simulink model "p10"  (R2020a)
settings: Solver=VariableStepAuto  StartTime=0.0  StopTime=10.0  RelTol=1e-3
model workspace (MAT data in the model file):
  A = 50
  Ad = 10
  B = 10
  C = 1389000
  H = 10000
  K = 2063000
  u = 1861.01
settings Model: Creator=a.kochnov  LastModifiedBy=a.kochnov

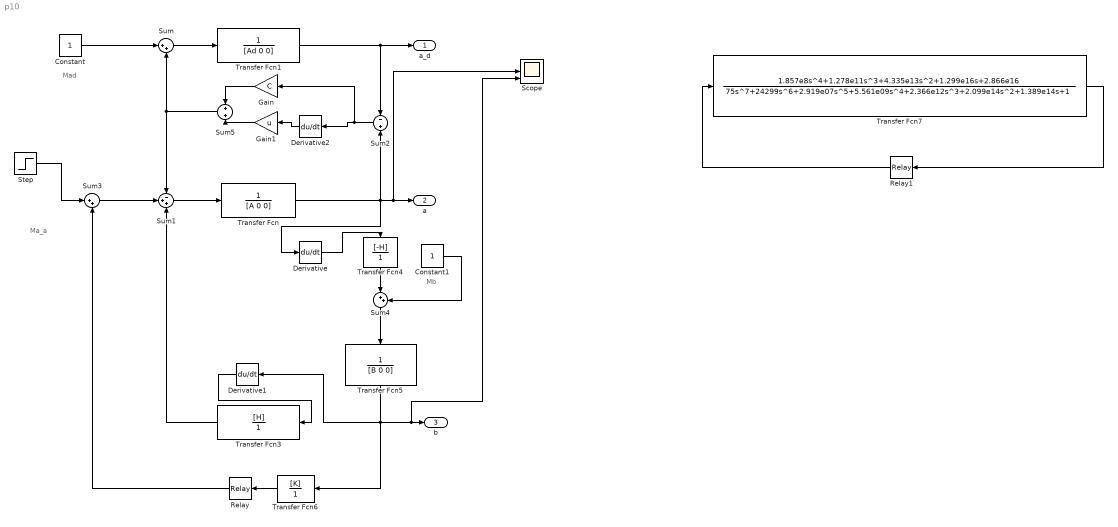
== system p10 ==
  note: Ma_a
  note: Mb
  note: Mad
  Constant : Constant
  Constant1 : Constant
  Derivative : Derivative
  Derivative1 : Derivative
  Derivative2 : Derivative
  Gain : Gain  Gain=C
  Gain1 : Gain  Gain=u
  Relay : Relay  OnSwitchValue=0  OffSwitchValue=0  OnOutputValue=10
  Relay1 : Relay  OnSwitchValue=0  OffSwitchValue=0
  Scope : Scope  NumInputPorts=3
  Step : Step  SampleTime=0
  Sum : Sum  Inputs=|++
  Sum1 : Sum  Inputs=-++
  Sum2 : Sum  Inputs=-|+
  Sum3 : Sum  Inputs=|++
  Sum4 : Sum  Inputs=|++
  Sum5 : Sum  Inputs=+|+
  Transfer Fcn : TransferFcn  Denominator=[A 0 0]
  Transfer Fcn1 : TransferFcn  Denominator=[Ad 0 0]
  Transfer Fcn3 : TransferFcn  Numerator=[H]  Denominator=[1]
  Transfer Fcn4 : TransferFcn  Numerator=[-H]  Denominator=1
  Transfer Fcn5 : TransferFcn  Denominator=[B 0 0]
  Transfer Fcn6 : TransferFcn  Numerator=[K]  Denominator=[1]
  Transfer Fcn7 : TransferFcn  Numerator=[1.857e8 1.278e11 4.335e13 1.299e16 2.866e16]  Denominator=[75 24299 2.919e07 5.561e09 2.366e12 2.099e14 1.389e14 1]
  a_d : Outport  SignalName=\alpha_d
  a : Outport  Port=2  SignalName=\alpha
  b : Outport  Port=3  SignalName=\\beta
  wires:
  Sum/1 -> Transfer Fcn1/1
  Sum1/1 -> Transfer Fcn/1
  Transfer Fcn1/1 -> a_d/1, Sum2/1
  Transfer Fcn/1 -> Derivative/1, Scope/2, a/1, Sum2/2
  Sum3/1 -> Sum1/2
  Transfer Fcn4/1 -> Sum4/1
  Constant/1 -> Sum/1
  Step/1 -> Sum3/1
  Constant1/1 -> Sum4/2
  Sum4/1 -> Transfer Fcn5/1
  Transfer Fcn5/1 -> Transfer Fcn6/1, Scope/3, b/1, Derivative1/1
  Transfer Fcn3/1 -> Sum1/3
  Transfer Fcn6/1 -> Relay/1
  Relay/1 -> Sum3/2
  Transfer Fcn7/1 -> Relay1/1
  Relay1/1 -> Transfer Fcn7/1
  Derivative/1 -> Transfer Fcn4/1
  Derivative1/1 -> Transfer Fcn3/1
  Derivative2/1 -> Gain1/1
  Sum2/1 -> Gain/1, Derivative2/1
  Gain/1 -> Sum5/1
  Gain1/1 -> Sum5/2
  Sum5/1 -> Sum1/1, Sum/2
